simulink model "bursting_linear"  (R2015a)
settings: Solver=ode45  StartTime=0.0  StopTime=3000  RelTol=1e-3
settings Model: Creator=ra428  LastModifiedBy=ra428

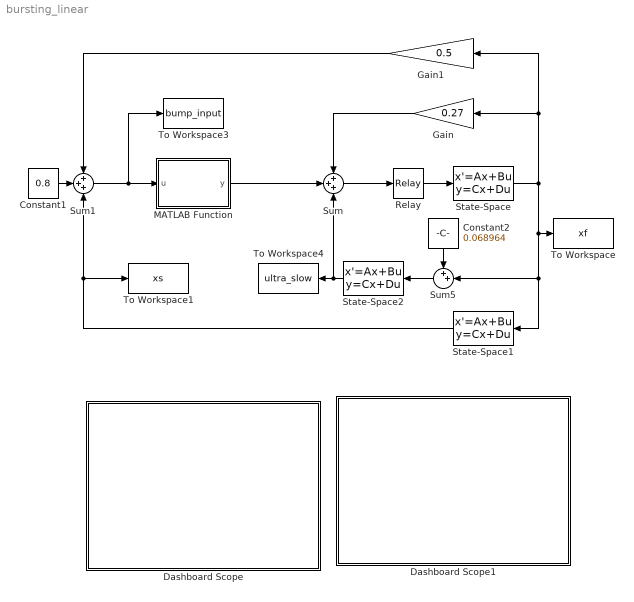
== system bursting_linear ==
  Constant1 : Constant  Value=0.8
  Constant2 : Constant  Value=0.068964
  Dashboard Scope : Subsystem  DialogController=hmiCreateDDGDialog  IsWebBlock=on  mask(MathWorksWebBlock){webBlockId=4bdcbcc0-e016-47be-a999-b9057f260784, webBlockType=sdiscope, ShowInitialText=on, HMISrcModelName=bursting_linear}
      mask prompts: webBlockId "WebBlock Id"; webBlockType "WebBlock Type"; HMISrcModelName "Source Model"
      mask Help: helpview([docroot '/mapfiles/simulink.map'], 'hmi_scope')
      mask Display:
      | if strcmp(get_param(bdroot(gcb),'BlockDiagramType'), 'library')
      |     image([(matlabroot) '/toolbox/simulink/hmi/icons/DashboardScope.png']);
      | end
  Dashboard Scope1 : Subsystem  DialogController=hmiCreateDDGDialog  IsWebBlock=on  mask(MathWorksWebBlock){webBlockId=a0db2e60-7909-413c-884d-ab9dd18d6060, webBlockType=sdiscope, ShowInitialText=on, HMISrcModelName=bursting_linear}
      mask prompts: webBlockId "WebBlock Id"; webBlockType "WebBlock Type"; HMISrcModelName "Source Model"
      mask Help: helpview([docroot '/mapfiles/simulink.map'], 'hmi_scope')
      mask Display:
      | if strcmp(get_param(bdroot(gcb),'BlockDiagramType'), 'library')
      |     image([(matlabroot) '/toolbox/simulink/hmi/icons/DashboardScope.png']);
      | end
  Gain : Gain  Gain=0.27
  Gain1 : Gain  Gain=0.5
  MATLAB Function : MATLAB Function  TreatAsAtomicUnit=on
  Relay : Relay  OffOutputValue=-1
  State-Space : StateSpace  A=-1000  B=1000  D=0  X0=-1.05
  State-Space1 : StateSpace  A=-1.686  B=1.686  D=0  X0=-1.05
  State-Space2 : StateSpace  A=-0.0026802  B=-0.0026802  D=0  X0=0
  Sum : Sum  Inputs=+++
  Sum1 : Sum  Inputs=+++
  Sum5 : Sum  Inputs=++|
  To Workspace : ToWorkspace  VariableName=xf  SaveFormat=Timeseries  SampleTime=-1
  To Workspace1 : ToWorkspace  VariableName=xs  SaveFormat=Timeseries  SampleTime=-1
  To Workspace3 : ToWorkspace  VariableName=bump_input  SaveFormat=Timeseries  SampleTime=-1
  To Workspace4 : ToWorkspace  VariableName=ultra_slow  SaveFormat=Timeseries  SampleTime=-1
  wires:
  Sum/1 -> Relay/1
  MATLAB Function/1(y) -> Sum/2
  Sum1/1 -> To Workspace3/1, MATLAB Function/1(u)
  Gain/1 -> Sum/1
  Gain1/1 -> Sum1/1
  Constant1/1 -> Sum1/2
  Relay/1 -> State-Space/1
  State-Space/1 -> State-Space1/1, Sum5/2, To Workspace/1, Gain/1, Gain1/1
  State-Space1/1 -> Sum1/3, To Workspace1/1
  Constant2/1 -> Sum5/1
  Sum5/1 -> State-Space2/1
  State-Space2/1 -> Sum/3, To Workspace4/1

== system bursting_linear/Dashboard Scope ==

== system bursting_linear/Dashboard Scope1 ==

== matlab function bursting_linear/MATLAB Function ==
  data: u input; y output
function y = fcn(u)
%#codegen
if (u < -2)
    y = -1;
elseif (u > 2)
    y = -1;
elseif and( u>=-2,u < 0)
    y = 0.5*u;
else
    y = -0.5*u;
end
